simulink model "DirectDrivePTO"  (R2014a)
settings: Solver=ode45  StartTime=0.0  StopTime=param.stop  FixedStep=0.0001  MaxStep=0.05  RelTol=1e-6
values from neighbouring files (symbols this model uses):
  lambda_fd = 8    [RunSimulation.m]
  lambda_sd_0 = 0    [RunSimulation.m]
  lambda_sq_0 = 0    [RunSimulation.m]
  Ls = 3/2*Lsinglephase    (= 0.285)    [RunSimulation.m]
  Rload = -200/1.7    (= -117.647058824)    [RunSimulation.m]
  Rs = 4.58    [RunSimulation.m]
  tau_p = 0.072    [RunSimulation.m]
  theta_d_0 = 0    [RunSimulation.m]
settings Model: Creator=brekken  LastModifiedBy=sor
settings DebuggingCC: MergeDetectMultiDrivingBlocksExec=error

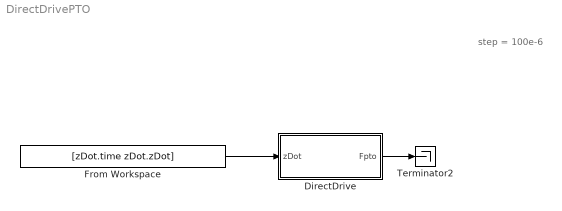
== system DirectDrivePTO ==
  note: step = 100e-6
  DirectDrive : Subsystem
  From Workspace : FromWorkspace  VariableName=[zDot.time zDot.zDot]  SampleTime=0  Interpolate=off  OutputAfterFinalValue=Holding final value
  Terminator2 : Terminator
  wires:
  From Workspace/1 -> DirectDrive/1(zDot)
  DirectDrive/1(Fpto) -> Terminator2/1

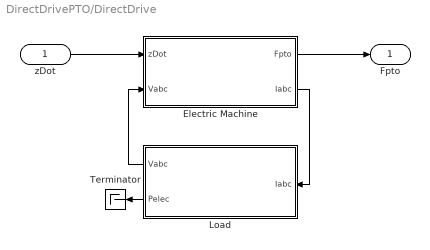
== system DirectDrivePTO/DirectDrive ==
  zDot : Inport
  "Electric Machine " : Subsystem
  Load : Subsystem
  Terminator : Terminator
  Fpto : Outport
  wires:
  "Electric Machine "/2(Iabc) -> Load/1(Iabc)
  Load/1(Vabc) -> "Electric Machine "/2(Vabc)
  zDot/1 -> "Electric Machine "/1(zDot)
  "Electric Machine "/1(Fpto) -> Fpto/1
  Load/2(Pelec) -> Terminator/1

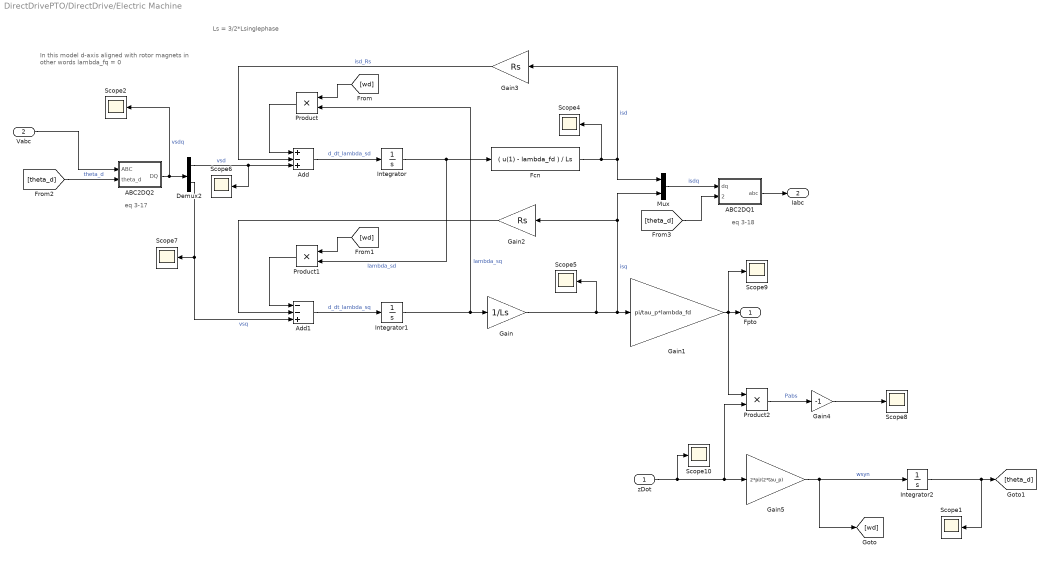
== system DirectDrivePTO/DirectDrive/Electric Machine  ==
  note: In this model d-axis aligned with rotor magnets
      | in other words lambda_fq = 0
  note: Ls = 3/2*Lsinglephase
  note: eq 3-17
  note: eq 3-18
  zDot : Inport
  Vabc : Inport  Port=2
  ABC2DQ1 : Subsystem
  ABC2DQ2 : Subsystem
  Add : Sum  Inputs=+-+
  Add1 : Sum  Inputs=--+
  Demux2 : Demux  Outputs=2
  Fcn : Fcn  Expr=( u(1) - lambda_fd ) / Ls
  Gain : Gain  Gain=1/Ls
  Gain1 : Gain  Gain=pi/tau_p*lambda_fd
  Gain2 : Gain  Gain=Rs
  Gain3 : Gain  Gain=Rs
  Gain4 : Gain  Gain=-1
  Gain5 : Gain  Gain=2*pi/(2*tau_p)
  Integrator : Integrator  InitialCondition=lambda_sd_0
  Integrator1 : Integrator  InitialCondition=lambda_sq_0
  Integrator2 : Integrator  InitialCondition=theta_d_0
  Mux : Mux  Inputs=2
  Product : Product  RndMeth=Zero
  Product1 : Product  RndMeth=Zero
  Product2 : Product
  Scope{1..2,4..10} (9 alike) : Scope
      Scope1 settings: SaveName=ScopeData7
      Scope10 settings: YMin=-3000  YMax=3000  SaveName=zDot
      Scope2 settings: YMin=-2.5e+27  YMax=3e+28  SaveName=ScopeData8
      Scope4 settings: YMin=-2.5e+27  YMax=3e+28  SaveName=ScopeData10
      Scope5 settings: YMin=-2.5e+27  YMax=3e+28  SaveName=ScopeData12
      Scope6 settings: YMin=-2.5e+27  YMax=3e+28  SaveName=ScopeData13
      Scope7 settings: YMin=-2.5e+27  YMax=3e+28  SaveName=ScopeData14
      Scope8 settings: YMin=-3000  YMax=3000  SaveName=Pabs
      Scope9 settings: YMin=-3000  YMax=3000  SaveName=Fpto
  Fpto : Outport
  Iabc : Outport  Port=2
  wires:
  Add/1 -> Integrator/1  "d_dt_lambda_sd"
  Integrator/1 -> Product1/2, Fcn/1  "lambda_sd"
  [wd] -> Product/1
  Fcn/1 -> Scope4/1, Gain3/1, Mux/1  "isd"
  Product/1 -> Add/1
  Add1/1 -> Integrator1/1  "d_dt_lambda_sq"
  Integrator1/1 -> Gain/1, Product/2  "lambda_sq"
  [wd] -> Product1/1
  Gain/1 -> Scope5/1, Gain1/1, Gain2/1, Mux/2  "isq"
  Product1/1 -> Add1/1
  Demux2/1 -> Scope6/1, Add/3  "vsd"
  Gain1/1 -> Scope9/1, Product2/1, Fpto/1
  Demux2/2 -> Scope7/1, Add1/3  "vsq"
  Vabc/1 -> ABC2DQ2/1(ABC)
  ABC2DQ2/1(DQ) -> Scope2/1, Demux2/1  "vsdq"
  Gain3/1 -> Add/2  "isd_Rs"
  Gain2/1 -> Add1/2
  [theta_d] -> ABC2DQ2/2(theta_d)  "theta_d"
  Mux/1 -> ABC2DQ1/1(dq)  "isdq"
  ABC2DQ1/1(abc) -> Iabc/1
  zDot/1 -> Scope10/1, Product2/2, Gain5/1
  Gain5/1 -> [wd], Integrator2/1  "wsyn"
  [theta_d] -> ABC2DQ1/2(theta_d)
  Integrator2/1 -> Scope1/1, [theta_d]
  Product2/1 -> Gain4/1  "Pabs"
  Gain4/1 -> Scope8/1

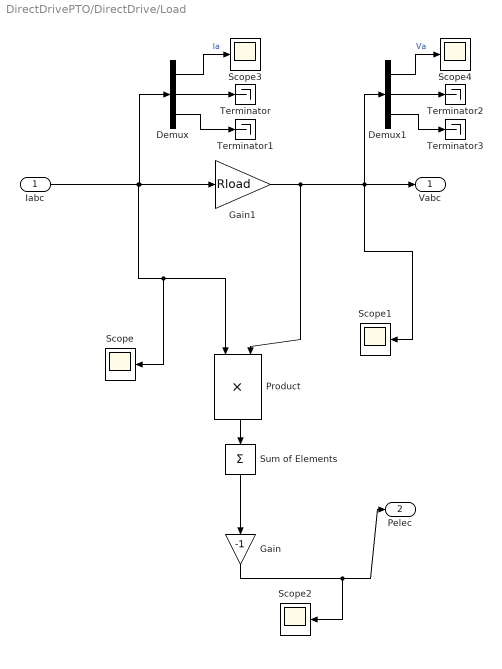
== system DirectDrivePTO/DirectDrive/Load ==
  Iabc : Inport
  Demux : Demux  Outputs=3
  Demux1 : Demux  Outputs=3
  Gain : Gain  Gain=-1
  Gain1 : Gain  Gain=Rload
  Product : Product
  Scope{,1..4} (5 alike) : Scope
      Scope settings: SaveName=Iabc
      Scope1 settings: SaveName=Vabc
      Scope2 settings: SaveName=Pelec
      Scope3 settings: SaveName=Ia
      Scope4 settings: SaveName=Va
  Sum of Elements : Sum  Inputs=+
  Terminator{,1..3} (4 alike) : Terminator
  Vabc : Outport
  Pelec : Outport  Port=2
  wires:
  Iabc/1 -> Product/1, Scope/1, Demux/1, Gain1/1
  Gain/1 -> Scope2/1, Pelec/1
  Gain1/1 -> Product/2, Demux1/1, Scope1/1, Vabc/1
  Product/1 -> Sum of Elements/1
  Sum of Elements/1 -> Gain/1
  Demux/1 -> Scope3/1  "Ia"
  Demux1/1 -> Scope4/1  "Va"
  Demux/2 -> Terminator/1
  Demux/3 -> Terminator1/1
  Demux1/2 -> Terminator2/1
  Demux1/3 -> Terminator3/1

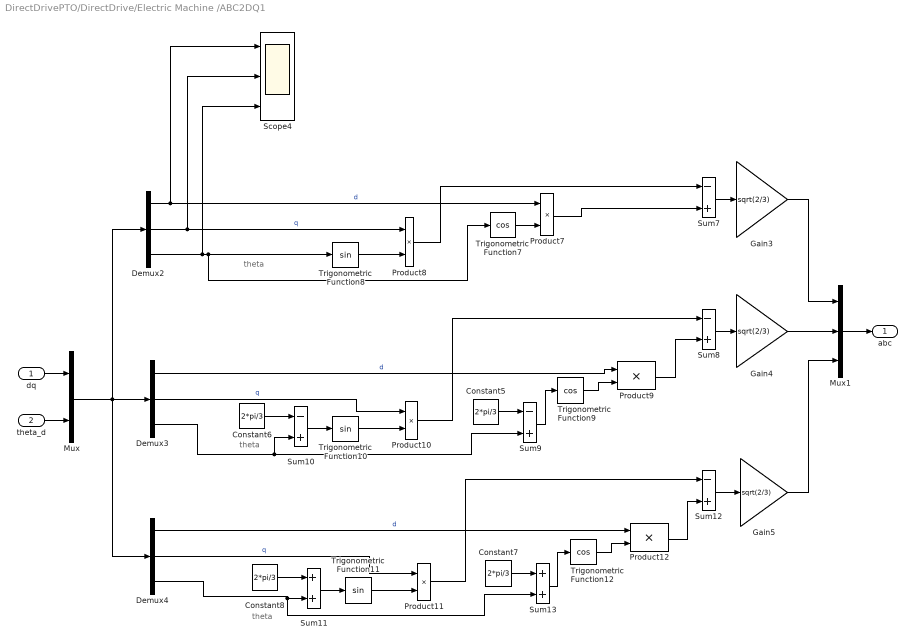
== system DirectDrivePTO/DirectDrive/Electric Machine /ABC2DQ1 ==
  note: theta
  note: theta
  note: theta
  dq : Inport
  theta_d : Inport  Port=2
  Constant{5..8} (4 alike) : Constant  Value=2*pi/3
  Demux2 : Demux  Outputs=3
  Demux3 : Demux  Outputs=3
  Demux4 : Demux  Outputs=3
  Gain3 : Gain  Gain=sqrt(2/3)  SaturateOnIntegerOverflow=on  OutDataTypeStr=Inherit: Same as input  ParamDataTypeStr=Inherit: Same as input
  Gain4 : Gain  Gain=sqrt(2/3)  SaturateOnIntegerOverflow=on  OutDataTypeStr=Inherit: Same as input  ParamDataTypeStr=Inherit: Same as input
  Gain5 : Gain  Gain=sqrt(2/3)  SaturateOnIntegerOverflow=on  OutDataTypeStr=Inherit: Same as input  ParamDataTypeStr=Inherit: Same as input
  Mux : Mux  Inputs=2
  Mux1 : Mux  Inputs=3
  Product{7..12} (6 alike) : Product  SaturateOnIntegerOverflow=on  InputSameDT=on  OutDataTypeStr=Inherit: Same as first input
  Scope4 : Scope  NumInputPorts=3
      settings: YMin=0~0~0  YMax=0.175~8.5~7  SaveName=ScopeData11
  Sum{7..10,12} (5 alike) : Sum  Inputs=-+  SaturateOnIntegerOverflow=on  InputSameDT=on  OutDataTypeStr=Inherit: Same as first input
  Sum11 : Sum  SaturateOnIntegerOverflow=on  InputSameDT=on  OutDataTypeStr=Inherit: Same as first input
  Sum13 : Sum  SaturateOnIntegerOverflow=on  InputSameDT=on  OutDataTypeStr=Inherit: Same as first input
  Trigonometric Function10 : Trigonometry
  Trigonometric Function11 : Trigonometry
  Trigonometric Function12 : Trigonometry  Operator=cos
  Trigonometric Function7 : Trigonometry  Operator=cos
  Trigonometric Function8 : Trigonometry
  Trigonometric Function9 : Trigonometry  Operator=cos
  abc : Outport
  wires:
  Mux1/1 -> abc/1
  dq/1 -> Mux/1
  theta_d/1 -> Mux/2
  Mux/1 -> Demux4/1, Demux2/1, Demux3/1
  Trigonometric Function7/1 -> Product7/2
  Demux2/1 -> Scope4/1, Product7/1  "d"
  Product7/1 -> Sum7/2
  Product8/1 -> Sum7/1
  Demux2/3 -> Scope4/3, Trigonometric Function8/1, Trigonometric Function7/1
  Demux2/2 -> Scope4/2, Product8/1  "q"
  Trigonometric Function9/1 -> Product9/2
  Demux3/1 -> Product9/1  "d"
  Product9/1 -> Sum8/2
  Product10/1 -> Sum8/1
  Demux3/3 -> Sum10/2, Sum9/2
  Trigonometric Function10/1 -> Product10/2
  Demux3/2 -> Product10/1  "q"
  Sum9/1 -> Trigonometric Function9/1
  Constant5/1 -> Sum9/1
  Sum10/1 -> Trigonometric Function10/1
  Constant6/1 -> Sum10/1
  Trigonometric Function12/1 -> Product12/2
  Demux4/1 -> Product12/1  "d"
  Product12/1 -> Sum12/2
  Product11/1 -> Sum12/1
  Demux4/3 -> Sum13/2, Sum11/2
  Trigonometric Function11/1 -> Product11/2
  Demux4/2 -> Product11/1  "q"
  Sum13/1 -> Trigonometric Function12/1
  Constant7/1 -> Sum13/1
  Sum11/1 -> Trigonometric Function11/1
  Constant8/1 -> Sum11/1
  Sum7/1 -> Gain3/1
  Sum8/1 -> Gain4/1
  Sum12/1 -> Gain5/1
  Gain3/1 -> Mux1/1
  Gain4/1 -> Mux1/2
  Gain5/1 -> Mux1/3
  Trigonometric Function8/1 -> Product8/2

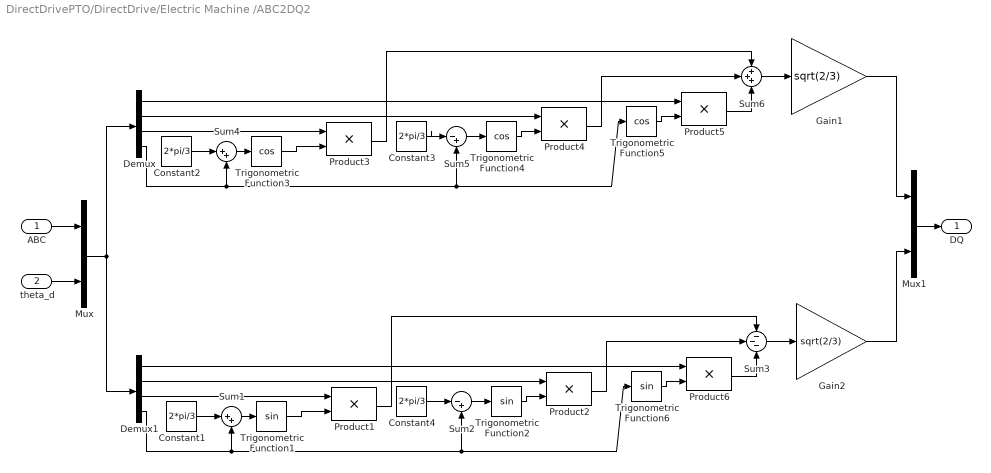
== system DirectDrivePTO/DirectDrive/Electric Machine /ABC2DQ2 ==
  ABC : Inport
  theta_d : Inport  Port=2
  Constant{1..4} (4 alike) : Constant  Value=2*pi/3
  Demux : Demux
  Demux1 : Demux
  Gain1 : Gain  Gain=sqrt(2/3)  SaturateOnIntegerOverflow=on  OutDataTypeStr=Inherit: Same as input  ParamDataTypeStr=Inherit: Same as input
  Gain2 : Gain  Gain=sqrt(2/3)  SaturateOnIntegerOverflow=on  OutDataTypeStr=Inherit: Same as input  ParamDataTypeStr=Inherit: Same as input
  Mux : Mux  Inputs=2
  Mux1 : Mux  Inputs=2
  Product{1..6} (6 alike) : Product  SaturateOnIntegerOverflow=on  InputSameDT=on  OutDataTypeStr=Inherit: Same as first input
  Sum1 : Sum  Inputs=|++  SaturateOnIntegerOverflow=on  InputSameDT=on  OutDataTypeStr=Inherit: Same as first input
  Sum2 : Sum  Inputs=|-+  SaturateOnIntegerOverflow=on  InputSameDT=on  OutDataTypeStr=Inherit: Same as first input
  Sum3 : Sum  Inputs=---  SaturateOnIntegerOverflow=on  InputSameDT=on  OutDataTypeStr=Inherit: Same as first input
  Sum4 : Sum  Inputs=|++  SaturateOnIntegerOverflow=on  InputSameDT=on  OutDataTypeStr=Inherit: Same as first input
  Sum5 : Sum  Inputs=|-+  SaturateOnIntegerOverflow=on  InputSameDT=on  OutDataTypeStr=Inherit: Same as first input
  Sum6 : Sum  Inputs=+++  SaturateOnIntegerOverflow=on  InputSameDT=on  OutDataTypeStr=Inherit: Same as first input
  Trigonometric Function1 : Trigonometry
  Trigonometric Function2 : Trigonometry
  Trigonometric Function3 : Trigonometry  Operator=cos
  Trigonometric Function4 : Trigonometry  Operator=cos
  Trigonometric Function5 : Trigonometry  Operator=cos
  Trigonometric Function6 : Trigonometry
  DQ : Outport
  wires:
  Mux1/1 -> DQ/1
  Product5/1 -> Sum6/3
  Constant2/1 -> Sum4/1
  Sum5/1 -> Trigonometric Function4/1
  Trigonometric Function4/1 -> Product4/2
  Trigonometric Function5/1 -> Product5/2
  Constant3/1 -> Sum5/1
  Sum6/1 -> Gain1/1
  Product3/1 -> Sum6/1
  Product4/1 -> Sum6/2
  Trigonometric Function3/1 -> Product3/2
  Gain1/1 -> Mux1/1
  ABC/1 -> Mux/1
  theta_d/1 -> Mux/2
  Demux/1 -> Product5/1
  Demux/2 -> Product4/1
  Demux/3 -> Product3/1
  Demux/4 -> Sum5/2, Trigonometric Function5/1, Sum4/2
  Mux/1 -> Demux/1, Demux1/1
  Sum4/1 -> Trigonometric Function3/1
  Product6/1 -> Sum3/3
  Constant1/1 -> Sum1/1
  Sum2/1 -> Trigonometric Function2/1
  Trigonometric Function2/1 -> Product2/2
  Trigonometric Function6/1 -> Product6/2
  Constant4/1 -> Sum2/1
  Sum3/1 -> Gain2/1
  Product1/1 -> Sum3/1
  Product2/1 -> Sum3/2
  Trigonometric Function1/1 -> Product1/2
  Gain2/1 -> Mux1/2
  Demux1/1 -> Product6/1
  Demux1/2 -> Product2/1
  Demux1/3 -> Product1/1
  Demux1/4 -> Sum1/2, Trigonometric Function6/1, Sum2/2
  Sum1/1 -> Trigonometric Function1/1
